simulink model "quarter_car_model"  (R2023a)
settings: Solver=FixedStepAuto  StartTime=0.0  StopTime=5  FixedStep=1e-3  RelTol=1e-3
values from neighbouring files (symbols this model uses):
  c_damper = 1500    [quarter_car_model_parameters.m]
  F0 = (m_s * g)-1814.85    (= 2109.15)    [quarter_car_model_parameters.m]
  k_spring = 35500    [quarter_car_model_parameters.m]
  k_tyre = 300000    [quarter_car_model_parameters.m]
  m_s = 400    [quarter_car_model_parameters.m]
  m_us = 30    [quarter_car_model_parameters.m]
  z0_tyre = (m_s + m_us) * g / k_tyre    (= 0.014061)    [quarter_car_model_parameters.m]
  z_r_type = 0    [quarter_car_model_parameters.m]
libraries: simulink x1
settings Model: Creator=Cassio de Freitas  LastModifiedBy=Cassio de Freitas
settings DataIOCC: ReturnWorkspaceOutputs=off

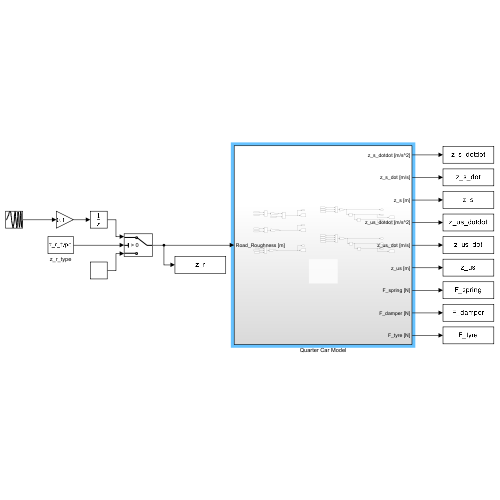
[thumbnail: Simulink's stored preview of the top-level diagram]
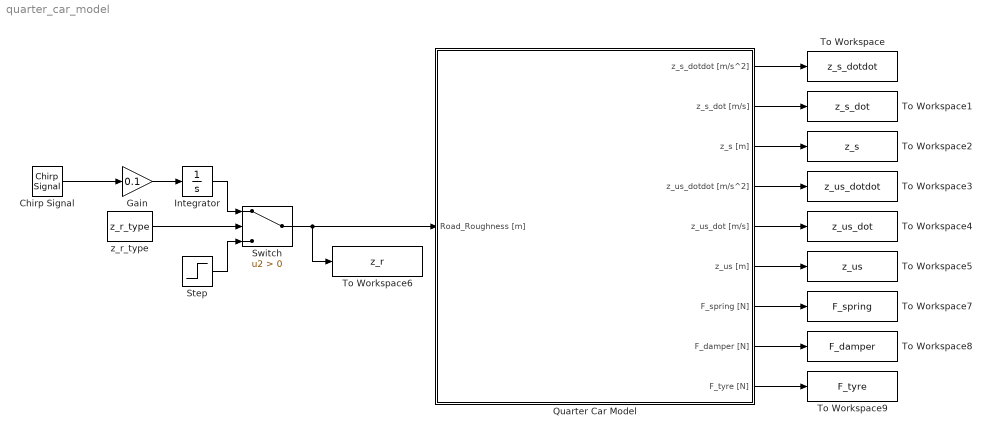
== system quarter_car_model ==
  Chirp Signal : simulink/Sources/Chirp Signal  f1=0.1  T=100  f2=50
  Gain : Gain  Gain=0.1
  Integrator : Integrator
  Quarter Car Model : Subsystem
  Step : Step  After=0.1  SampleTime=1e-3
  Switch : Switch  Criteria=u2 > Threshold  SaturateOnIntegerOverflow=off  InputSameDT=off
  To Workspace : ToWorkspace  VariableName=z_s_dotdot  SaveFormat=Timeseries  SampleTime=-1
  To Workspace1 : ToWorkspace  VariableName=z_s_dot  SaveFormat=Timeseries  SampleTime=-1
  To Workspace2 : ToWorkspace  VariableName=z_s  SaveFormat=Timeseries  SampleTime=-1
  To Workspace3 : ToWorkspace  VariableName=z_us_dotdot  SaveFormat=Timeseries  SampleTime=-1
  To Workspace4 : ToWorkspace  VariableName=z_us_dot  SaveFormat=Timeseries  SampleTime=-1
  To Workspace5 : ToWorkspace  VariableName=z_us  SaveFormat=Timeseries  SampleTime=-1
  To Workspace6 : ToWorkspace  VariableName=z_r  SaveFormat=Timeseries  SampleTime=-1
  To Workspace7 : ToWorkspace  VariableName=F_spring  SaveFormat=Timeseries  SampleTime=-1
  To Workspace8 : ToWorkspace  VariableName=F_damper  SaveFormat=Timeseries  SampleTime=-1
  To Workspace9 : ToWorkspace  VariableName=F_tyre  SaveFormat=Timeseries  SampleTime=-1
  z_r_type : Constant  Value=z_r_type
  wires:
  Quarter Car Model/1(z_s_dotdot [m/s^2]) -> To Workspace/1
  Quarter Car Model/2(z_s_dot [m/s]) -> To Workspace1/1
  Quarter Car Model/3(z_s [m]) -> To Workspace2/1
  Quarter Car Model/4(z_us_dotdot [m/s^2]) -> To Workspace3/1
  Quarter Car Model/5(z_us_dot [m/s]) -> To Workspace4/1
  Quarter Car Model/6(z_us [m]) -> To Workspace5/1
  Gain/1 -> Integrator/1
  Chirp Signal/1 -> Gain/1
  Integrator/1 -> Switch/1
  Switch/1 -> To Workspace6/1, Quarter Car Model/1(Road_Roughness [m])
  Step/1 -> Switch/3
  z_r_type/1 -> Switch/2
  Quarter Car Model/9(F_tyre [N]) -> To Workspace9/1
  Quarter Car Model/8(F_damper [N]) -> To Workspace8/1
  Quarter Car Model/7(F_spring [N]) -> To Workspace7/1

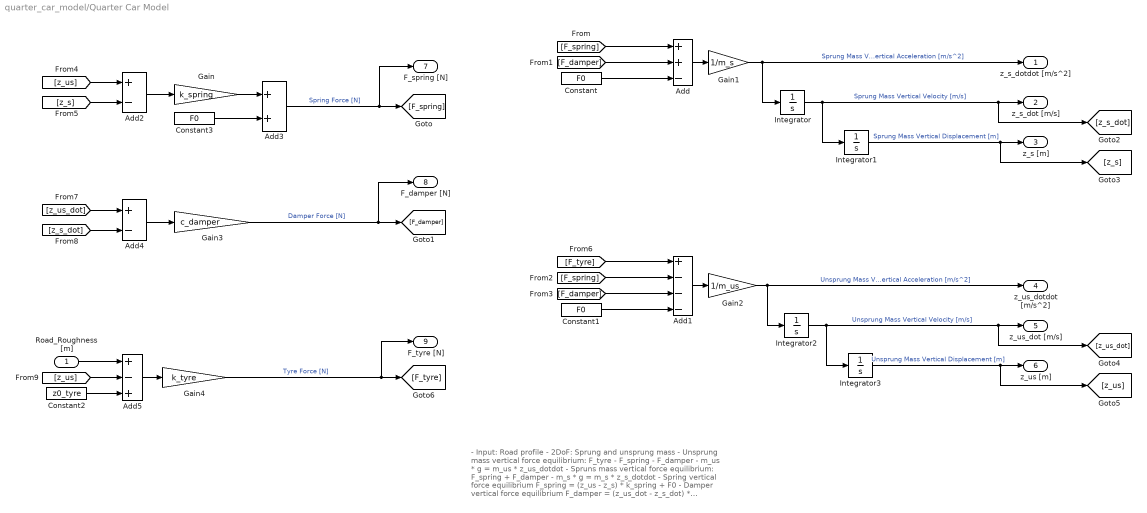
== system quarter_car_model/Quarter Car Model ==
  note: - Input: Road profile
      |
      | - 2DoF: Sprung and unsprung mass
      |
      | - Unsprung mass vertical force equilibrium:
      | F_tyre - F_spring - F_damper - m_us * g = m_us * z_us_dotdot
      |
      | - Spruns mass vertical force equilibrium:
      | F_spring + F_damper - m_s * g = m_s * z_s_dotdot
      |
      | - Spring vertical force equilibrium
      | F_spring = (z_us - z_s) * k_spring + F0
      |
      | - Damper vertical force equilibrium
      | F_damper = (z_us_dot - z_s_dot) * c_damper
      |
      | - Tyre vertical force equilibrium
      | F_tyre = (z_r - z_us +z0_tyre) * k_tyre
  Road_Roughness [m] : Inport
  Add : Sum  Inputs=++-
  Add1 : Sum  Inputs=+---
  Add2 : Sum  Inputs=+-
  Add3 : Sum
  Add4 : Sum  Inputs=+-
  Add5 : Sum  Inputs=+-+
  Constant : Constant  Value=F0
  Constant1 : Constant  Value=F0
  Constant2 : Constant  Value=z0_tyre
  Constant3 : Constant  Value=F0
  Gain : Gain  Gain=k_spring
  Gain1 : Gain  Gain=1/m_s
  Gain2 : Gain  Gain=1/m_us
  Gain3 : Gain  Gain=c_damper
  Gain4 : Gain  Gain=k_tyre
  Integrator{,1..3} (4 alike) : Integrator
  z_s_dotdot [m/s^2] : Outport
  z_s_dot [m/s] : Outport  Port=2
  z_s [m] : Outport  Port=3
  z_us_dotdot [m/s^2] : Outport  Port=4
  z_us_dot [m/s] : Outport  Port=5
  z_us [m] : Outport  Port=6
  F_spring [N] : Outport  Port=7
  F_damper [N] : Outport  Port=8
  F_tyre [N] : Outport  Port=9
  wires:
  Add/1 -> Gain1/1
  Integrator/1 -> Integrator1/1, [z_s_dot], z_s_dot [m/s]/1  "Sprung Mass Vertical Velocity [m/s]"
  Integrator1/1 -> [z_s], z_s [m]/1  "Sprung Mass Vertical Displacement [m]"
  [F_spring] -> Add/1
  [F_damper] -> Add/2
  Constant/1 -> Add/3
  Add1/1 -> Gain2/1
  Constant1/1 -> Add1/4
  [F_damper] -> Add1/3
  [F_spring] -> Add1/2
  Gain1/1 -> Integrator/1, z_s_dotdot [m/s^2]/1  "Sprung Mass Vertical Acceleration [m/s^2]"
  Gain2/1 -> Integrator2/1, z_us_dotdot [m/s^2]/1  "Unsprung Mass Vertical Acceleration [m/s^2]"
  [z_us] -> Add2/1
  [z_s] -> Add2/2
  Add2/1 -> Gain/1
  Gain/1 -> Add3/1
  Constant3/1 -> Add3/2
  Add3/1 -> F_spring [N]/1, [F_spring]  "Spring Force [N]"
  Add4/1 -> Gain3/1
  [z_s_dot] -> Add4/2
  [z_us_dot] -> Add4/1
  Gain3/1 -> F_damper [N]/1, [F_damper]  "Damper Force [N]"
  Integrator3/1 -> z_us [m]/1, [z_us]  "Unsprung Mass Vertical Displacement [m]"
  Integrator2/1 -> z_us_dot [m/s]/1, [z_us_dot], Integrator3/1  "Unsprung Mass Vertical Velocity [m/s]"
  [z_us] -> Add5/2
  Constant2/1 -> Add5/3
  Road_Roughness [m]/1 -> Add5/1
  Add5/1 -> Gain4/1
  Gain4/1 -> F_tyre [N]/1, [F_tyre]  "Tyre Force [N]"
  [F_tyre] -> Add1/1
